simulink model "simple_math_operation"  (R2024b)
settings: Solver=ode3  StartTime=0.0  StopTime=10.0  FixedStep=1  RelTol=1e-3
settings Model: Creator=balaj  LastModifiedBy=balaj

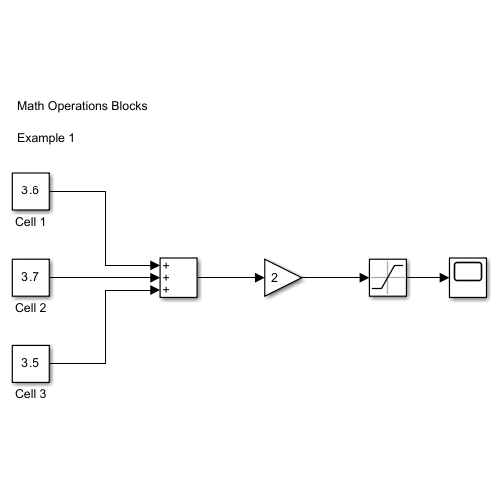
[thumbnail: Simulink's stored preview of the top-level diagram]
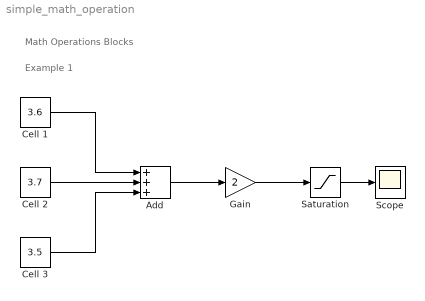
== system simple_math_operation ==
  note: Math Operations Blocks
  note: Example 1
  Add : Sum  Inputs=+++
  Cell 1 : Constant  Value=3.6  SampleTime=1
  Cell 2 : Constant  Value=3.7  SampleTime=1
  Cell 3 : Constant  Value=3.5  SampleTime=1
  Gain : Gain  Gain=2
  Saturation : Saturate  UpperLimit=12  LowerLimit=0
  Scope : Scope
  wires:
  Cell 1/1 -> Add/1
  Cell 2/1 -> Add/2
  Cell 3/1 -> Add/3
  Add/1 -> Gain/1
  Gain/1 -> Saturation/1
  Saturation/1 -> Scope/1
